simulink model "pid_controller"  (R2020a)
settings: Solver=VariableStepAuto  StartTime=0.0  StopTime=20  RelTol=1e-3
settings Model: Creator=USER  LastModifiedBy=USER

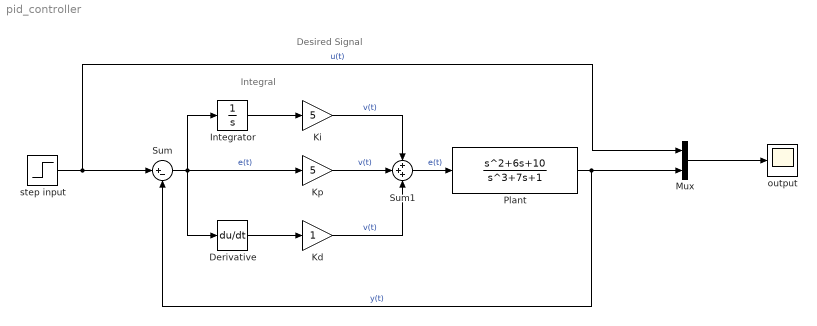
== system pid_controller ==
  note: Desired Signal
  note: Integral
  Derivative : Derivative
  Integrator : Integrator
  Kd : Gain
  Ki : Gain  Gain=5
  Kp : Gain  Gain=5
  Mux : Mux  Inputs=2
  Plant : TransferFcn  Numerator=[1 6 10]  Denominator=[1 0 7 1]
  Sum : Sum  Inputs=|+-
  Sum1 : Sum  Inputs=+++
  output : Scope
  step input : Step  SampleTime=0
  wires:
  step input/1 -> Mux/1, Sum/1  "u(t)"
  Plant/1 -> Mux/2, Sum/2  "y(t)"
  Sum/1 -> Derivative/1, Integrator/1, Kp/1  "e(t)"
  Kp/1 -> Sum1/2  "v(t)"
  Mux/1 -> output/1
  Ki/1 -> Sum1/1  "v(t)"
  Sum1/1 -> Plant/1  "e(t)"
  Integrator/1 -> Ki/1
  Derivative/1 -> Kd/1
  Kd/1 -> Sum1/3  "v(t)"
